simulink library "NAV420DecodeLib_LowLevel"  (Simulink 7.3)
settings: Solver=ode45  StartTime=0.0  StopTime=10.0  RelTol=1e-3
libraries: simulink x7
settings Model: Creator=djulzz  LastModifiedBy=djulzz

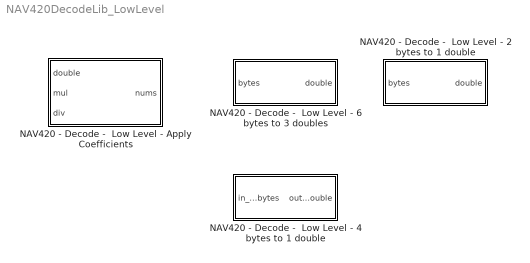
== system NAV420DecodeLib_LowLevel ==
  NAV420 - Decode -  Low Level - 2 bytes to 1 double : Subsystem
  NAV420 - Decode -  Low Level - 4 bytes to 1 double : Subsystem
  NAV420 - Decode -  Low Level - 6 bytes to 3 doubles : Subsystem
  NAV420 - Decode -  Low Level - Apply Coefficients : Subsystem

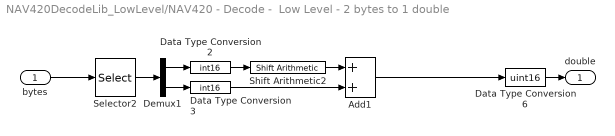
== system NAV420DecodeLib_LowLevel/NAV420 - Decode -  Low Level - 2 bytes to 1 double ==
  bytes : Inport
  Add1 : Sum  OutDataType=fixdt(1, 16)  OutScaling=2^-10
  Data Type Conversion2 : DataTypeConversion  OutDataTypeMode=int16  OutDataType=fixdt(1, 16)  OutScaling=2^0  OutDataTypeStr=int16
  Data Type Conversion3 : DataTypeConversion  OutDataTypeMode=int16  OutDataType=fixdt(1, 16)  OutScaling=2^0  OutDataTypeStr=int16
  Data Type Conversion6 : DataTypeConversion  OutDataTypeMode=uint16  OutDataType=fixdt(1, 16)  OutScaling=2^0  OutDataTypeStr=uint16
  Demux1 : Demux  Outputs=2
  Selector2 : Selector  InputPortWidth=2  IndexOptions=Index vector (dialog)  Indices=[1 2]  OutputSizes=1
  Shift Arithmetic2 : simulink/Logic and Bit Operations/Shift Arithmetic  SystemSampleTime=-1  nBitShiftRight=-8  nBinPtShiftRight=0
  double : Outport  DataType=uint16  OutDataTypeStr=uint16
  wires:
  bytes/1 -> Selector2/1
  Selector2/1 -> Demux1/1
  Demux1/1 -> Data Type Conversion2/1
  Demux1/2 -> Data Type Conversion3/1
  Data Type Conversion2/1 -> Shift Arithmetic2/1
  Data Type Conversion3/1 -> Add1/2
  Shift Arithmetic2/1 -> Add1/1
  Data Type Conversion6/1 -> double/1
  Add1/1 -> Data Type Conversion6/1

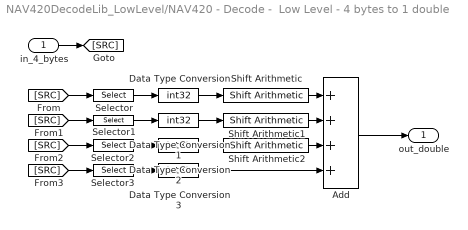
== system NAV420DecodeLib_LowLevel/NAV420 - Decode -  Low Level - 4 bytes to 1 double ==
  in_4_bytes : Inport  DataType=uint8  OutDataType=fixdt(1, 16)  OutScaling=2^0  OutDataTypeStr=uint8
  Add : Sum  Inputs=++++  AccumDataTypeStr=int32  OutDataTypeMode=double  OutDataType=fixdt(1, 16)  OutScaling=2^-10  OutDataTypeStr=double
  Data Type Conversion{,1..3} (4 alike) : DataTypeConversion  OutDataTypeMode=int32  OutDataType=fixdt(1, 16)  OutScaling=2^0  OutDataTypeStr=int32
  Selector : Selector  InputPortWidth=4  IndexOptions=Index vector (dialog)  Indices=[1]  OutputSizes=1
  Selector1 : Selector  InputPortWidth=4  IndexOptions=Index vector (dialog)  Indices=[2]  OutputSizes=1
  Selector2 : Selector  InputPortWidth=4  IndexOptions=Index vector (dialog)  Indices=[3]  OutputSizes=1
  Selector3 : Selector  InputPortWidth=4  IndexOptions=Index vector (dialog)  Indices=[4]  OutputSizes=1
  Shift Arithmetic : simulink/Logic and Bit Operations/Shift Arithmetic  SystemSampleTime=-1  nBitShiftRight=-24  nBinPtShiftRight=0
  Shift Arithmetic1 : simulink/Logic and Bit Operations/Shift Arithmetic  SystemSampleTime=-1  nBitShiftRight=-16  nBinPtShiftRight=0
  Shift Arithmetic2 : simulink/Logic and Bit Operations/Shift Arithmetic  SystemSampleTime=-1  nBitShiftRight=-8  nBinPtShiftRight=0
  out_double : Outport  OutDataType=fixdt(1, 16)  OutScaling=2^0
  wires:
  in_4_bytes/1 -> [SRC]
  [SRC] -> Selector/1
  [SRC] -> Selector1/1
  [SRC] -> Selector2/1
  [SRC] -> Selector3/1
  Selector/1 -> Data Type Conversion/1
  Data Type Conversion/1 -> Shift Arithmetic/1
  Selector1/1 -> Data Type Conversion1/1
  Data Type Conversion1/1 -> Shift Arithmetic1/1
  Selector2/1 -> Data Type Conversion2/1
  Data Type Conversion2/1 -> Shift Arithmetic2/1
  Shift Arithmetic/1 -> Add/1
  Shift Arithmetic1/1 -> Add/2
  Shift Arithmetic2/1 -> Add/3
  Data Type Conversion3/1 -> Add/4
  Selector3/1 -> Data Type Conversion3/1
  Add/1 -> out_double/1

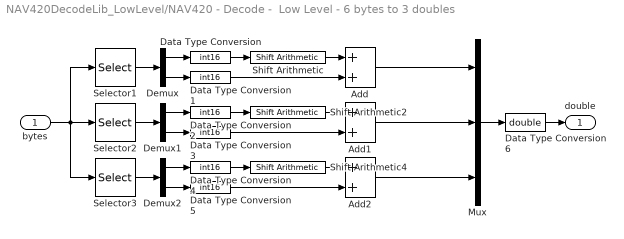
== system NAV420DecodeLib_LowLevel/NAV420 - Decode -  Low Level - 6 bytes to 3 doubles ==
  bytes : Inport
  Add : Sum  OutDataType=fixdt(1, 16)  OutScaling=2^-10
  Add1 : Sum  OutDataType=fixdt(1, 16)  OutScaling=2^-10
  Add2 : Sum  OutDataType=fixdt(1, 16)  OutScaling=2^-10
  Data Type Conversion{,1..5} (6 alike) : DataTypeConversion  OutDataTypeMode=int16  OutDataType=fixdt(1, 16)  OutScaling=2^0  OutDataTypeStr=int16
  Data Type Conversion6 : DataTypeConversion  OutDataTypeMode=double  OutDataType=fixdt(1, 16)  OutScaling=2^0  OutDataTypeStr=double
  Demux : Demux  Outputs=2
  Demux1 : Demux  Outputs=2
  Demux2 : Demux  Outputs=2
  Mux : Mux  Inputs=3
  Selector1 : Selector  InputPortWidth=6  IndexOptions=Index vector (dialog)  Indices=[1 2]  OutputSizes=1
  Selector2 : Selector  InputPortWidth=6  IndexOptions=Index vector (dialog)  Indices=[3 4]  OutputSizes=1
  Selector3 : Selector  InputPortWidth=6  IndexOptions=Index vector (dialog)  Indices=[5 6]  OutputSizes=1
  Shift Arithmetic : simulink/Logic and Bit Operations/Shift Arithmetic  SystemSampleTime=-1  nBitShiftRight=-8  nBinPtShiftRight=0
  Shift Arithmetic2 : simulink/Logic and Bit Operations/Shift Arithmetic  SystemSampleTime=-1  nBitShiftRight=-8  nBinPtShiftRight=0
  Shift Arithmetic4 : simulink/Logic and Bit Operations/Shift Arithmetic  SystemSampleTime=-1  nBitShiftRight=-8  nBinPtShiftRight=0
  double : Outport
  wires:
  bytes/1 -> Selector3/1, Selector1/1, Selector2/1
  Selector1/1 -> Demux/1
  Demux/1 -> Data Type Conversion/1
  Demux/2 -> Data Type Conversion1/1
  Data Type Conversion/1 -> Shift Arithmetic/1
  Data Type Conversion1/1 -> Add/2
  Shift Arithmetic/1 -> Add/1
  Selector2/1 -> Demux1/1
  Demux1/1 -> Data Type Conversion2/1
  Demux1/2 -> Data Type Conversion3/1
  Data Type Conversion2/1 -> Shift Arithmetic2/1
  Data Type Conversion3/1 -> Add1/2
  Shift Arithmetic2/1 -> Add1/1
  Selector3/1 -> Demux2/1
  Demux2/1 -> Data Type Conversion4/1
  Demux2/2 -> Data Type Conversion5/1
  Data Type Conversion4/1 -> Shift Arithmetic4/1
  Data Type Conversion5/1 -> Add2/2
  Shift Arithmetic4/1 -> Add2/1
  Add2/1 -> Mux/3
  Add1/1 -> Mux/2
  Add/1 -> Mux/1
  Mux/1 -> Data Type Conversion6/1
  Data Type Conversion6/1 -> double/1

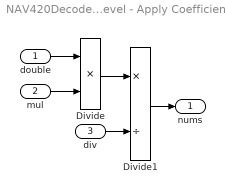
== system NAV420DecodeLib_LowLevel/NAV420 - Decode -  Low Level - Apply Coefficients ==
  double : Inport
  mul : Inport  Port=2
  div : Inport  Port=3
  Divide : Product  Inputs=**  OutDataType=fixdt(1, 16)  OutScaling=2^-10
  Divide1 : Product  Inputs=*/  OutDataType=fixdt(1, 16)  OutScaling=2^-10
  nums : Outport
  wires:
  Divide/1 -> Divide1/1
  double/1 -> Divide/1
  mul/1 -> Divide/2
  Divide1/1 -> nums/1
  div/1 -> Divide1/2
